simulink model "sltestBaselineBasicExample"  (R2017a)
settings: Solver=ode45  StartTime=0.0  StopTime=10.0  RelTol=1e-3  EnableMultiTasking=on
PostLoadFcn:
  | gain2_var = 2;
CloseFcn:
  | clear gain2_var;
Description:
  | sltestBaselineBasicExample model.
  | This model has two outputs which can be used for baseline comparison. A variable is loaded in the model callbacks which can be modified from the workspace to try different baseline scenarios.
settings Model: Creator=The MathWorks, Inc.  LastModifiedBy=The MathWorks, Inc.
settings DataIOCC: LimitDataPoints=on  SaveFormat=Array
settings OptimizationCC: LifeSpan=inf
settings DebuggingCC: SFUnexpectedBacktrackingDiag=warning  SFNoUnconditionalDefaultTransitionDiag=warning  SFExecutionAtInitializationDiag=none
settings HardwareCC: ProdBitPerPointer=32  ProdBitPerSizeT=32  ProdBitPerPtrDiffT=32  ProdLargestAtomicFloat=None  ProdIntDivRoundTo=Undefined  ProdEndianess=Unspecified  ProdWordSize=32  ProdHWDeviceType=32-bit Generic
settings ModelReferenceCC: PropagateSignalLabelsOutOfModel=off
settings GRTTargetCC: TargetLangStandard=C89/C90 (ANSI)  GeneratePreprocessorConditionals=Disable all
settings ConfigComp: CovMetricSettings=dw  CovHtmlReporting=on  CovSaveCumulativeToWorkspaceVar=on  CovSaveSingleToWorkspaceVar=on  CovExternalEMLEnable=off  CovSFcnEnable=off

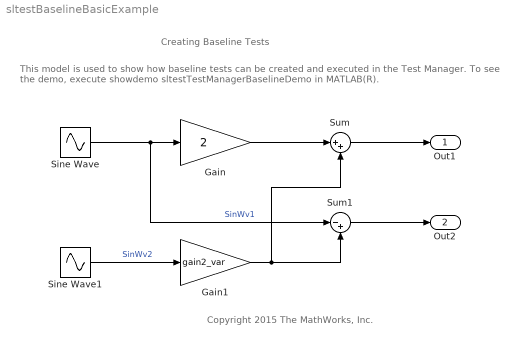
== system sltestBaselineBasicExample ==
  note: This model is used to show how baseline tests can be created and executed in the Test Manager.
      | To see the demo, execute showdemo sltestTestManagerBaselineDemo in MATLAB(R).
  note: Creating Baseline Tests
  note: Copyright 2015 The MathWorks, Inc.
  Gain : Gain  Gain=2
  Gain1 : Gain  Gain=gain2_var
  Sine Wave : Sin  SampleTime=0
  Sine Wave1 : Sin  Phase=pi  SampleTime=0
  Sum : Sum  Inputs=|++
  Sum1 : Sum  Inputs=|-+
  Out1 : Outport
  Out2 : Outport  Port=2
  wires:
  Sine Wave/1 -> Gain/1, Sum1/1  "SinWv1"
  Gain/1 -> Sum/1
  Sum/1 -> Out1/1
  Sine Wave1/1 -> Gain1/1  "SinWv2"
  Sum1/1 -> Out2/1
  Gain1/1 -> Sum/2, Sum1/2
